simulink model "stm32f0_clcd_2lines_demo"  (Simulink 7.3)
settings: Solver=ode3  SolverMode=SingleTasking  StartTime=0.0  StopTime=10.0  RelTol=1e-3
PreLoadFcn:
  | waijung.modelPreload; % Required for working with Waijung Blockset. Do not remove.
undefined symbols (not defined in the file): LQFP48, STM32F072CB
libraries: simulink x1, waijung_crc_lib x1, stm32f0_device_config_lib x1
CloseFcn:
  | waijung.modelClose; % Required for working with Waijung Blockset. Do not remove.
settings Model: Creator=Krisada  LastModifiedBy=Krisada
settings OptimizationCC: OptimizeModelRefInitCode=on  LifeSpan=1
settings HardwareCC: ProdEndianess=LittleEndian  ProdHWDeviceType=ARM Compatible->Cortex - M0  TargetEndianess=LittleEndian  TargetHWDeviceType=ARM Compatible->Cortex - M0
settings RTWCC: SystemTargetFile=stm32f0.tlc  GenerateMakefile=off  TemplateMakefile=ert_default_tmf  Description=STM32F0 Target  ProcessScript=stm32f0_make_rtw_hook
settings CodeAppCC: IgnoreCustomStorageClasses=off
settings STFCustomTargetCC: ModelReferenceCompliant=off  CombineOutputUpdateFcns=on  ERTCustomFileBanners=on  SupportContinuousTime=off  SupportNonInlinedSFcns=off  SystemTargetFile=stm32f0.tlc
settings ERTTargetCC: MultiwordLength=2048  ModelReferenceCompliant=off  ParMdlRefBuildCompliant=off  CompOptLevelCompliant=off  ERTFirstTimeCompliant=off  ModelStepFunctionPrototypeControlCompliant=off  CPPClassGenCompliant=off  InlinedParameterPlacement=NonHierarchical  ERTSrcFileBannerTemplate=stm32f0_code_template.cgt  ERTHdrFileBannerTemplate=stm32f0_code_template.cgt  ERTDataSrcFileTemplate=stm32f0_code_template.cgt  ERTDataHdrFileTemplate=stm32f0_code_template.cgt  ERTCustomFileTemplate=stm32f0_file_process.tlc

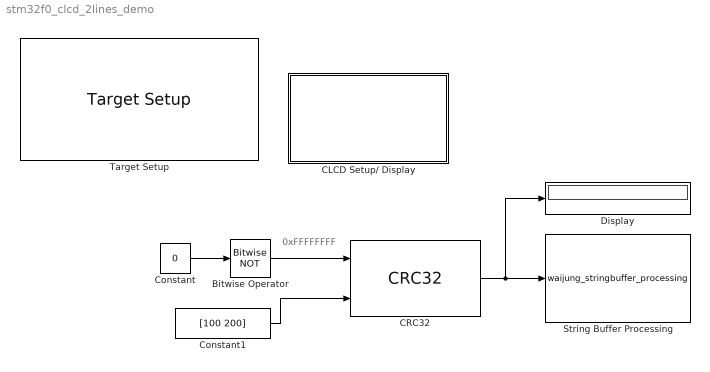
== system stm32f0_clcd_2lines_demo ==
  note: 0xFFFFFFFF
  Bitwise Operator : simulink/Logic and Bit Operations/Bitwise Operator  logicop=NOT  UseBitMask=off  BitMask=bin2dec('11011001')  BitMaskRealWorld=Stored Integer
  CLCD Setup/ Display : Subsystem
  CRC32 : waijung_crc_lib/CRC32  conf=<empty>  sampletime=inf  enablecustomportlabel=off  cinputportlabel=0  portpinstr=0  blockid=CRC32  inputporttype=[7 7]  inputportwidth=[1 -1]  inputportlabel={'Initial','Value'}  outputporttype=[7]  outputportwidth=[]  outputportlabel={'Output'}  compat=0  optionstring="[\"Param1\",\"Param1\"]"
  Constant : Constant  Value=0  OutDataTypeMode=uint32  OutDataType=fixdt(1, 16)  OutScaling=2^0  OutDataTypeStr=uint32
  Constant1 : Constant  Value=[100 200]  OutDataTypeMode=uint32  OutDataType=fixdt(1, 16)  OutScaling=2^0  OutDataTypeStr=uint32
  Display : Display
      settings: Format=hex (Stored Integer)
  String Buffer Processing : S-Function  FunctionName=waijung_stringbuffer_processing  Parameters=configuration,varname,sformat,porttypes,portcount,inputtypearray,outputtypearray,sampletime,sampletimestr,blockid  EnableBusSupport=off  mask(waijung_stringbuffer_processing){configuration=sprintf, storagename=line2, sformat='0x%X', enableoutput=off, varname=CLCDSetupDisplayVolatileDataStorage1_line2, inputtypearray=[1 -1], outputtypearray=[0], porttypes=["uint32_t"], portcount=1, sampletime=-1, sampletimestr=0.01, blockid=StringBufferProcessing}
      mask prompts: configuration "Function"; storagename "String buffer"; sformat "Printf format"; enableoutput "Enable output status"; varname "Variable name"; inputtypearray "Input type array"; outputtypearray "Output type array"; porttypes "Port type list"; portcount "Port type count"; sampletime "Sample time (sec)"; sampletimestr "Compiled sample time (sec) in string"
      mask help:
      | This block implements string processing, sprintf/ sscanf command.
      | Supported format:
      | %u, %i, %o, %x: uint32
      | %d: int32
      | %e, %g, %f: single
      | %c: int8
      |
      | Status:
      |  0: Failed.
      |  Non-zero: Success.
      mask init:
      | waijung_stringbuffer_processing_callback('init');
      mask Help: web(fullfile(waijungdocroot,'String_Buffer_Processing.htm'))
      mask StyleString: popup(sprintf|sscanf),popup(line1|line2|<output>),edit,checkbox,edit,edit,edit,edit,edit,edit,edit,edit
      mask CallbackString: waijung_stringbuffer_processing_callback('configuration');||waijung_stringbuffer_processing_callback('sformat');|waijung_stringbuffer_processing_callback('enableoutput');||||||waijung_stringbuffer_processing_callback('sampletime');|waijung_stringbuffer_processing_callback('sampletimestr');|waijung_stringbuffer_processing_callback('blockid');
      mask Display: text(0.5, 0.5, '[ sprintf ]\nBuffer: line2\nTs (sec): 0.01','ver','middle','hor','center');port_label('input', 1,'%X');
  Target Setup : stm32f0_device_config_lib/Target Setup  Priority=100  compiler=GNU ARM  previous_compiler=GNU ARM  mcu=STM32F072CB (LQFP48)  mcustr=STM32F072CB  stdlib=STM32F072  clockconfig=FiO MOTE-ST Default (HSEOSC-8MHz/HCLK-48MHz)  system_stm32f0xx_c_path=F:\trunk\targets\stm32f0_target\stm32f0\utils\STM32F0xx_AN4055\stm32f0_default\hse8mhz_pll_hclk48mhz  showmemoryconfiguration=on  stacksize=0x400  heapsize=0x200  enableautocompiledownload=on  fullchiperase=off  programmerinterface=aMG USB Connect  editctrlstr=on  compilercontrolstr=$(patsubst %, -I%, .) -mcpu=cortex-m0 -mthumb -mabi=aapcs -Wall -O3 -mfloat-abi=soft -ffunction-sections -fdata-sections -fno-strict-aliasing -fno-builtin --short-enums  assemblercontrolstr=$(patsubst %, -I%, .) -mcpu=cortex-m0 -mtune=cortex-m0 -mthumb -Wall -O3 -Wa,-amhls=$(<:.s=.lst) -D__STACK_SIZE=$(STACK_SIZE) -D__HEAP_SIZE=$(HEAP_SIZE)  linkercontrolstr="-T$(LD_SCRIPT) -Wl,-Map=$(MAP),--cref,--no-warn-mismatch -mcpu=cortex-m0 -mthumb  -Wall -O3 -mabi=aapcs -lc -specs=nosys.specs"  runafterdownload=on  execprofile=None  profileruart=3  profilerbaud=500000  profilertxpin=Not used  profilerinitstr=0.01,48000000,480000,500000,0  manualsetsampletime=on  sampletime=0.01  blockid=TargetSetup  systickreloadvalue=480000  hseval=8000000  lastprofileruart=3  hclk=48000000  flashorigin=0x8000000  flashlength=128k  ramorigin=0x20000000  ramlength=16k  useextram=off
  wires:
  Constant/1 -> Bitwise Operator/1
  Bitwise Operator/1 -> CRC32/1
  Constant1/1 -> CRC32/2
  CRC32/1 -> String Buffer Processing/1, Display/1

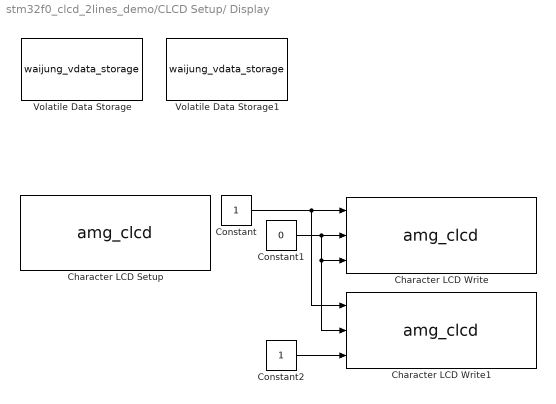
== system stm32f0_clcd_2lines_demo/CLCD Setup/ Display ==
  Character LCD Setup : S-Function  FunctionName=amg_clcd  Parameters=module,configuration,inputtypearray,outputtypearray,confstr,sampletime,sampletimestr,blockid  EnableBusSupport=off  mask(amg_clcd){configuration=Setup, module=1, model=amg CLCD Std, interface=4-bits, linecount=4, columncount=16, gpiotype=Push-pull, controlport=A, control_rs=8, control_rw=11, control_en=12, dataport=B, data0=10, data1=11, data2=12, data3=13, usestringbuffer=off, stringbuffer=<empty>, varname=, inputtypearray=[0], outputtypearray=[0], confstr=["4","4","16","PP","A","8","12","11","","B","","","","","10","11","12","13","0","","1","1","0","0","0","0","0","0","0","stm32f0"], sampletime=-1, sampletimestr=0.01, blockid=CLCDSetupDisplayCharacterLCDSetup}
      mask prompts: model "LCD model:"; linecount "Number of lines (2 or 4):"; columncount "Number of columns (16 or 20):"; gpiotype "GPIO Output type:"; controlport "GPIO control port:"; control_rs "GPIO control pin, RS:"; control_rw "GPIO control pin, RW:"; control_en "GPIO control pin, EN:"; dataport "GPIO data D[7:4] port"; data0 "GPIO data pin, D4:"; data1 "GPIO data pin, D5:"; data2 "GPIO data pin, D6:"; data3 "GPIO data pin, D7:"; usestringbuffer "Use string buffer"; stringbuffer "String buffer"; varname "Variable name"; inputtypearray "Input type array"; outputtypearray "Output type array"; confstr "Configuration string"; sampletime "Sample time (sec)"; sampletimestr "Compiled sample time (sec) in string"
      mask init:
      | amg_clcd_callback('init');
      mask Help: web(fullfile(waijungdocroot,'amg_clcd_setup.htm'), '-browser')
      mask StyleString: popup(Setup|Transaction),popup(1|2|3|4),popup(amg CLCD Std),popup(4-bits),edit,edit,popup(Push-pull|Open-drain),popup(A|B|C|D|E|F|G|H|I),popup(0|1|2|3|4|5|6|7|8|9|10|11|12|13|14|15),popup(0|1|2|3|4|5|6|7|8|9|10|11|12|13|14|15),popup(0|1|2|3|4|5|6|7|8|9|10|11|12|13|14|15),popup(A|B|C|D|E|F|G|H|I),popup(0|1|2|3|4|5|6|7|8|9|10|11|12|13|14|15),popup(0|1|2|3|4|5|6|7|8|9|10|11|12|13|14|15),popup(0|1|2|3|4|5|6|7|8|9|10|11|12|13|14|15),popup(0|1|2|3|4|5|6|7|8|9|10|11|12|13|14|15),checkbox,popup(<empty>),edit,edit,edit,edit,edit,edit,edit
      mask CallbackString: amg_clcd_callback('configuration');||||||||||||||||amg_clcd_callback('usestringbuffer');||amg_clcd_callback('varname');|||amg_clcd_callback('confstr');|amg_clcd_callback('sampletime');|amg_clcd_callback('sampletimestr');|amg_clcd_callback('blockid');
      mask Display: text(0.5, 0.5, 'Module: CLCD1 (Setup)\nInterface: 4-bits\nCntrl: A8/A11/A12\nD[7:4]: B10/B11/B12/B13\nTs (sec): 0.01','ver','middle','hor','center');
  Character LCD Write : S-Function  FunctionName=amg_clcd  Parameters=module,configuration,inputtypearray,outputtypearray,confstr,sampletime,sampletimestr,blockid  EnableBusSupport=off  mask(amg_clcd){configuration=Transaction, module=1, model=amg CLCD Std, interface=4-bits, linecount=4, columncount=20, gpiotype=Push-pull, controlport=E, control_rs=15, control_rw=13, control_en=11, dataport=A, data0=7, data1=5, data2=3, data3=1, usestringbuffer=on, stringbuffer=line1, varname=CLCDSetupDisplayVolatileDataStorage_line1, inputtypearray=[3 -1 -1 -1], outputtypearray=[0], confstr=["4","4","20","PP","E","15","11","13","","A","","","","","7","5","3","1","1","CLCDSetupDisplayVolatileDataStorage_line1","1","0","0","0","1","0","0","0","0","stm32f0"], sampletime=-1, sampletimestr=0.01, blockid=CLCDSetupDisplayCharacterLCDWrite}
      mask prompts: model "LCD model:"; linecount "Number of lines:"; columncount "Number of columns:"; gpiotype "GPIO Output type:"; controlport "GPIO control port:"; control_rs "GPIO control pin, RS:"; control_rw "GPIO control pin, RW:"; control_en "GPIO control pin, EN:"; dataport "GPIO data D[7:4] port"; data0 "GPIO data pin, D4:"; data1 "GPIO data pin, D5:"; data2 "GPIO data pin, D6:"; data3 "GPIO data pin, D7:"; usestringbuffer "Use string buffer"; stringbuffer "String buffer"; varname "Variable name"; inputtypearray "Input type array"; outputtypearray "Output type array"; confstr "Configuration string"; sampletime "Sample time (sec)"; sampletimestr "Compiled sample time (sec) in string"
      mask help:
      | Note for cmd:
      | 1 - Clear specified LCD line display before write data to LCD.
      | Otherwise (e.g. 0) - Write data without clearing LCD Line.
      |
      | Position:
      | x = 0, First Character (from left to right)
      | y = 0, Top Line
      mask init:
      | amg_clcd_callback('init');
      mask Help: web(fullfile(waijungdocroot,'amg_clcd_write.htm'), '-browser')
      mask StyleString: popup(Setup|Transaction),popup(1|2|3|4),popup(amg CLCD Std),popup(4-bits),edit,edit,popup(Push-pull|Open-drain),popup(A|B|C|D|E|F|G|H|I),popup(0|1|2|3|4|5|6|7|8|9|10|11|12|13|14|15),popup(0|1|2|3|4|5|6|7|8|9|10|11|12|13|14|15),popup(0|1|2|3|4|5|6|7|8|9|10|11|12|13|14|15),popup(A|B|C|D|E|F|G|H|I),popup(0|1|2|3|4|5|6|7|8|9|10|11|12|13|14|15),popup(0|1|2|3|4|5|6|7|8|9|10|11|12|13|14|15),popup(0|1|2|3|4|5|6|7|8|9|10|11|12|13|14|15),popup(0|1|2|3|4|5|6|7|8|9|10|11|12|13|14|15),checkbox,popup(line1|line2),edit,edit,edit,edit,edit,edit,edit
      mask CallbackString: amg_clcd_callback('configuration');||||||||||||||||amg_clcd_callback('usestringbuffer');||amg_clcd_callback('varname');|||amg_clcd_callback('confstr');|amg_clcd_callback('sampletime');|amg_clcd_callback('sampletimestr');|amg_clcd_callback('blockid');
      mask Display: text(0.5, 0.5, 'Module: CLCD1 (Write)\nBuffer: line1\nTs (sec): 0.01','ver','middle','hor','center');port_label('input', 1,'cmd');port_label('input', 2,'xpos');port_label('input', 3,'ypos');
  Character LCD Write1 : S-Function  FunctionName=amg_clcd  Parameters=module,configuration,inputtypearray,outputtypearray,confstr,sampletime,sampletimestr,blockid  EnableBusSupport=off  mask(amg_clcd){configuration=Transaction, module=1, model=amg CLCD Std, interface=4-bits, linecount=4, columncount=20, gpiotype=Push-pull, controlport=E, control_rs=15, control_rw=13, control_en=11, dataport=A, data0=7, data1=5, data2=3, data3=1, usestringbuffer=on, stringbuffer=line2, varname=CLCDSetupDisplayVolatileDataStorage1_line2, inputtypearray=[3 -1 -1 -1], outputtypearray=[0], confstr=["4","4","20","PP","E","15","11","13","","A","","","","","7","5","3","1","1","CLCDSetupDisplayVolatileDataStorage1_line2","1","0","0","0","1","0","0","0","0","stm32f0"], sampletime=-1, sampletimestr=0.01, blockid=CLCDSetupDisplayCharacterLCDWrite1}
      mask prompts: model "LCD model:"; linecount "Number of lines:"; columncount "Number of columns:"; gpiotype "GPIO Output type:"; controlport "GPIO control port:"; control_rs "GPIO control pin, RS:"; control_rw "GPIO control pin, RW:"; control_en "GPIO control pin, EN:"; dataport "GPIO data D[7:4] port"; data0 "GPIO data pin, D4:"; data1 "GPIO data pin, D5:"; data2 "GPIO data pin, D6:"; data3 "GPIO data pin, D7:"; usestringbuffer "Use string buffer"; stringbuffer "String buffer"; varname "Variable name"; inputtypearray "Input type array"; outputtypearray "Output type array"; confstr "Configuration string"; sampletime "Sample time (sec)"; sampletimestr "Compiled sample time (sec) in string"
      mask help:
      | Note for cmd:
      | 1 - Clear specified LCD line display before write data to LCD.
      | Otherwise (e.g. 0) - Write data without clearing LCD Line.
      |
      | Position:
      | x = 0, First Character (from left to right)
      | y = 0, Top Line
      mask init:
      | amg_clcd_callback('init');
      mask Help: web(fullfile(waijungdocroot,'amg_clcd_write.htm'), '-browser')
      mask StyleString: popup(Setup|Transaction),popup(1|2|3|4),popup(amg CLCD Std),popup(4-bits),edit,edit,popup(Push-pull|Open-drain),popup(A|B|C|D|E|F|G|H|I),popup(0|1|2|3|4|5|6|7|8|9|10|11|12|13|14|15),popup(0|1|2|3|4|5|6|7|8|9|10|11|12|13|14|15),popup(0|1|2|3|4|5|6|7|8|9|10|11|12|13|14|15),popup(A|B|C|D|E|F|G|H|I),popup(0|1|2|3|4|5|6|7|8|9|10|11|12|13|14|15),popup(0|1|2|3|4|5|6|7|8|9|10|11|12|13|14|15),popup(0|1|2|3|4|5|6|7|8|9|10|11|12|13|14|15),popup(0|1|2|3|4|5|6|7|8|9|10|11|12|13|14|15),checkbox,popup(line1|line2),edit,edit,edit,edit,edit,edit,edit
      mask CallbackString: amg_clcd_callback('configuration');||||||||||||||||amg_clcd_callback('usestringbuffer');||amg_clcd_callback('varname');|||amg_clcd_callback('confstr');|amg_clcd_callback('sampletime');|amg_clcd_callback('sampletimestr');|amg_clcd_callback('blockid');
      mask Display: text(0.5, 0.5, 'Module: CLCD1 (Write)\nBuffer: line2\nTs (sec): 0.01','ver','middle','hor','center');port_label('input', 1,'cmd');port_label('input', 2,'xpos');port_label('input', 3,'ypos');
  Constant : Constant  OutDataType=fixdt(1, 16)  OutScaling=2^0
  Constant1 : Constant  Value=0  OutDataType=fixdt(1, 16)  OutScaling=2^0
  Constant2 : Constant  OutDataType=fixdt(1, 16)  OutScaling=2^0
  Volatile Data Storage : S-Function  FunctionName=waijung_vdata_storage  Parameters=storagetype,storagename,initval,varname,buffersize,initvalstring,sampletime,sampletimestr,blockid,storagetypestr  EnableBusSupport=off  mask(waijung_vdata_storage){storagetype=string, definevolatile=off, storagename=line1, initval=0, varname=CLCDSetupDisplayVolatileDataStorage_line1, buffersize=20, initvalstring='STM32F0 Target', webintegration=Disable, weboutputformat='%s', webcgicallback=(void*)0, laststoragetype=string, sampletime=-1, sampletimestr=0.01, blockid=CLCDSetupDisplayVolatileDataStorage, storagetypestr=char}
      mask prompts: storagetype "Storage Type"; definevolatile "Define with "volatile" keyword"; storagename "Storage Name (must be a valid variable name)"; initval "Initial value (Apply at Power on Reset only)"; varname "Variable name"; buffersize "Size (bytes)"; initvalstring "Initial value (Apply at Power on Reset only)"; webintegration "Web CGI varget/varset integration"; weboutputformat "Web CGI varget output format"; webcgicallback "Web CGI varset callback"; laststoragetype "Last selected Storage Type"; sampletime "Sample time (sec)"; sampletimestr "Compiled sample time (sec) in string"; storagetypestr "Type string"
      mask help:
      | This block implements a volatile Data Storage.
      |
      | Web CGI varset/varget integratiopn:
      | Enable - In webserver application, allow remote access via http.
      | Disable - Variable is use in local only.
      mask init:
      | waijung_vdata_storage_callback('init');
      mask Help: web(fullfile(waijungdocroot,'Volatile_Data_Storage.htm'))
      mask StyleString: popup(double|single|uint32|int32|uint16|int16|uint8|int8|string),checkbox,edit,edit,edit,edit,edit,popup(Disable|ReadOnly|Write/ Read|ReadOnly with KeyValuePair|Write/ Read with KeyValuePair),edit,edit,popup(double|single|uint32|int32|uint16|int16|uint8|int8|string),edit,edit,edit,edit
      mask CallbackString: waijung_vdata_storage_callback('storagetype');||waijung_vdata_storage_callback('storagename');|waijung_vdata_storage_callback('initval');|waijung_vdata_storage_callback('varname');||waijung_vdata_storage_callback('initvalstring');|waijung_vdata_storage_callback('webintegration');|waijung_vdata_storage_callback('weboutputformat');|||waijung_vdata_storage_callback('sampletime');|waijung_vdata_storage_callback('sampletimestr');|waijung_vdata_storage_callback('blockid');|
      mask Display: text(0.5, 0.5, 'Name: line1\nType: string','ver','middle','hor','center')
  Volatile Data Storage1 : S-Function  FunctionName=waijung_vdata_storage  Parameters=storagetype,storagename,initval,varname,buffersize,initvalstring,sampletime,sampletimestr,blockid,storagetypestr  EnableBusSupport=off  mask(waijung_vdata_storage){storagetype=string, definevolatile=off, storagename=line2, initval=0, varname=CLCDSetupDisplayVolatileDataStorage1_line2, buffersize=20, initvalstring='000', webintegration=Disable, weboutputformat='%s', webcgicallback=(void*)0, laststoragetype=string, sampletime=-1, sampletimestr=0.01, blockid=CLCDSetupDisplayVolatileDataStorage1, storagetypestr=char}
      mask prompts: storagetype "Storage Type"; definevolatile "Define with "volatile" keyword"; storagename "Storage Name (must be a valid variable name)"; initval "Initial value (Apply at Power on Reset only)"; varname "Variable name"; buffersize "Size (bytes)"; initvalstring "Initial value (Apply at Power on Reset only)"; webintegration "Web CGI varget/varset integration"; weboutputformat "Web CGI varget output format"; webcgicallback "Web CGI varset callback"; laststoragetype "Last selected Storage Type"; sampletime "Sample time (sec)"; sampletimestr "Compiled sample time (sec) in string"; storagetypestr "Type string"
      mask help:
      | This block implements a volatile Data Storage.
      |
      | Web CGI varset/varget integratiopn:
      | Enable - In webserver application, allow remote access via http.
      | Disable - Variable is use in local only.
      mask init:
      | waijung_vdata_storage_callback('init');
      mask Help: web(fullfile(waijungdocroot,'Volatile_Data_Storage.htm'))
      mask StyleString: popup(double|single|uint32|int32|uint16|int16|uint8|int8|string),checkbox,edit,edit,edit,edit,edit,popup(Disable|ReadOnly|Write/ Read|ReadOnly with KeyValuePair|Write/ Read with KeyValuePair),edit,edit,popup(double|single|uint32|int32|uint16|int16|uint8|int8|string),edit,edit,edit,edit
      mask CallbackString: waijung_vdata_storage_callback('storagetype');||waijung_vdata_storage_callback('storagename');|waijung_vdata_storage_callback('initval');|waijung_vdata_storage_callback('varname');||waijung_vdata_storage_callback('initvalstring');|waijung_vdata_storage_callback('webintegration');|waijung_vdata_storage_callback('weboutputformat');|||waijung_vdata_storage_callback('sampletime');|waijung_vdata_storage_callback('sampletimestr');|waijung_vdata_storage_callback('blockid');|
      mask Display: text(0.5, 0.5, 'Name: line2\nType: string','ver','middle','hor','center')
  wires:
  Constant/1 -> Character LCD Write/1, Character LCD Write1/1
  Constant1/1 -> Character LCD Write/2, Character LCD Write/3, Character LCD Write1/2
  Constant2/1 -> Character LCD Write1/3
